simulink model "parallel_8_prediction_and_cost_function"  (R2022a)
settings: Solver=FixedStepDiscrete  StartTime=0.0  StopTime=10.0  RelTol=1e-3
undefined symbols (not defined in the file or in its folder): f_c, L_d, L_q, L_x, L_y, p, psi_pm, R_ph
libraries: hdlsllib x10
(part 2 of 2)

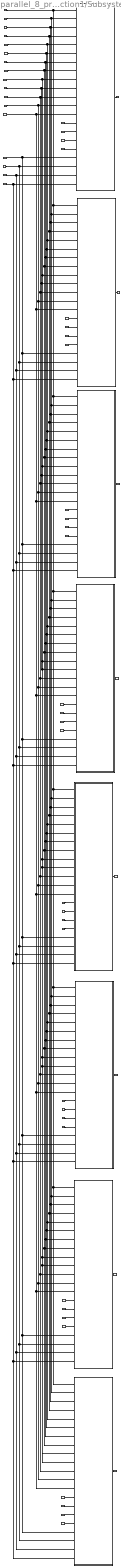
== system parallel_8_prediction_and_cost_function/Prediction_and_cost_function1/Subsystem ==
  d_phase_voltage_per_switching_state : Inport
  q_phase_voltage_per_switching_state : Inport  Port=2
  x_phase_voltage_per_switching_state : Inport  Port=3
  y_phase_voltage_per_switching_state : Inport  Port=4
  d_phase_voltage_per_switching_state1 : Inport  Port=5
  q_phase_voltage_per_switching_state1 : Inport  Port=6
  x_phase_voltage_per_switching_state1 : Inport  Port=7
  y_phase_voltage_per_switching_state1 : Inport  Port=8
  d_phase_voltage_per_switching_state2 : Inport  Port=9
  q_phase_voltage_per_switching_state2 : Inport  Port=10
  x_phase_voltage_per_switching_state2 : Inport  Port=11
  y_phase_voltage_per_switching_state2 : Inport  Port=12
  d_phase_voltage_per_switching_state3 : Inport  Port=13
  q_phase_voltage_per_switching_state3 : Inport  Port=14
  x_phase_voltage_per_switching_state3 : Inport  Port=15
  y_phase_voltage_per_switching_state3 : Inport  Port=16
  d_phase_voltage_per_switching_state4 : Inport  Port=17
  q_phase_voltage_per_switching_state4 : Inport  Port=18
  x_phase_voltage_per_switching_state4 : Inport  Port=19
  y_phase_voltage_per_switching_state4 : Inport  Port=20
  d_phase_voltage_per_switching_state5 : Inport  Port=21
  q_phase_voltage_per_switching_state5 : Inport  Port=22
  x_phase_voltage_per_switching_state5 : Inport  Port=23
  y_phase_voltage_per_switching_state5 : Inport  Port=24
  d_phase_voltage_per_switching_state6 : Inport  Port=25
  q_phase_voltage_per_switching_state6 : Inport  Port=26
  x_phase_voltage_per_switching_state6 : Inport  Port=27
  y_phase_voltage_per_switching_state6 : Inport  Port=28
  d_phase_voltage_per_switching_state7 : Inport  Port=29
  q_phase_voltage_per_switching_state7 : Inport  Port=30
  x_phase_voltage_per_switching_state7 : Inport  Port=31
  y_phase_voltage_per_switching_state7 : Inport  Port=32
  SampleTime_div_Ld15 : Inport  Port=33
  SampleTime_div_Lq15 : Inport  Port=34
  SampleTime_div_Lx15 : Inport  Port=35
  SampleTime_div_Ly15 : Inport  Port=36
  id_k_16 : Inport  Port=37
  iq_k_16 : Inport  Port=38
  ix_k_16 : Inport  Port=39
  iy_k_16 : Inport  Port=40
  Rs15 : Inport  Port=41
  omega_el15 : Inport  Port=42
  Lq15 : Inport  Port=43
  Ld15 : Inport  Port=44
  psiPM15 : Inport  Port=45
  id_ref15 : Inport  Port=46
  iq_ref15 : Inport  Port=47
  ix_ref15 : Inport  Port=48
  iy_ref15 : Inport  Port=49
  MATLAB Function10 : MATLAB Function  TreatAsAtomicUnit=on  SystemSampleTime=1/100000000
  MATLAB Function11 : MATLAB Function  TreatAsAtomicUnit=on  SystemSampleTime=1/100000000
  MATLAB Function12 : MATLAB Function  TreatAsAtomicUnit=on  SystemSampleTime=1/100000000
  MATLAB Function13 : MATLAB Function  TreatAsAtomicUnit=on  SystemSampleTime=1/100000000
  MATLAB Function14 : MATLAB Function  TreatAsAtomicUnit=on  SystemSampleTime=1/100000000
  MATLAB Function15 : MATLAB Function  TreatAsAtomicUnit=on  SystemSampleTime=1/100000000
  MATLAB Function8 : MATLAB Function  TreatAsAtomicUnit=on  SystemSampleTime=1/100000000
  MATLAB Function9 : MATLAB Function  TreatAsAtomicUnit=on  SystemSampleTime=1/100000000
  J : Outport
  J1 : Outport  Port=2
  J2 : Outport  Port=3
  J3 : Outport  Port=4
  J4 : Outport  Port=5
  J5 : Outport  Port=6
  J6 : Outport  Port=7
  J7 : Outport  Port=8
  wires:
  q_phase_voltage_per_switching_state1/1 -> MATLAB Function14/15(q_phase_voltage_per_switching_state)
  SampleTime_div_Ld15/1 -> MATLAB Function8/1(SampleTime_div_Ld), MATLAB Function9/1(SampleTime_div_Ld), MATLAB Function10/1(SampleTime_div_Ld), MATLAB Function11/1(SampleTime_div_Ld), MATLAB Function12/1(SampleTime_div_Ld), MATLAB Function13/1(SampleTime_div_Ld), MATLAB Function14/1(SampleTime_div_Ld), MATLAB Function15/1(SampleTime_div_Ld)
  Rs15/1 -> MATLAB Function8/9(Rs), MATLAB Function9/9(Rs), MATLAB Function10/9(Rs), MATLAB Function11/9(Rs), MATLAB Function12/9(Rs), MATLAB Function13/9(Rs), MATLAB Function14/9(Rs), MATLAB Function15/9(Rs)
  y_phase_voltage_per_switching_state/1 -> MATLAB Function15/17(y_phase_voltage_per_switching_state)
  Lq15/1 -> MATLAB Function8/11(Lq), MATLAB Function9/11(Lq), MATLAB Function10/11(Lq), MATLAB Function11/11(Lq), MATLAB Function12/11(Lq), MATLAB Function13/11(Lq), MATLAB Function14/11(Lq), MATLAB Function15/11(Lq)
  MATLAB Function11/1(J) -> J4/1
  y_phase_voltage_per_switching_state2/1 -> MATLAB Function13/17(y_phase_voltage_per_switching_state)
  d_phase_voltage_per_switching_state1/1 -> MATLAB Function14/14(d_phase_voltage_per_switching_state)
  x_phase_voltage_per_switching_state1/1 -> MATLAB Function14/16(x_phase_voltage_per_switching_state)
  y_phase_voltage_per_switching_state7/1 -> MATLAB Function8/17(y_phase_voltage_per_switching_state)
  iy_ref15/1 -> MATLAB Function8/21(iy_ref), MATLAB Function9/21(iy_ref), MATLAB Function10/21(iy_ref), MATLAB Function11/21(iy_ref), MATLAB Function12/21(iy_ref), MATLAB Function13/21(iy_ref), MATLAB Function14/21(iy_ref), MATLAB Function15/21(iy_ref)
  omega_el15/1 -> MATLAB Function8/10(omega_el), MATLAB Function9/10(omega_el), MATLAB Function10/10(omega_el), MATLAB Function11/10(omega_el), MATLAB Function12/10(omega_el), MATLAB Function13/10(omega_el), MATLAB Function14/10(omega_el), MATLAB Function15/10(omega_el)
  psiPM15/1 -> MATLAB Function8/13(psiPM), MATLAB Function9/13(psiPM), MATLAB Function10/13(psiPM), MATLAB Function11/13(psiPM), MATLAB Function12/13(psiPM), MATLAB Function13/13(psiPM), MATLAB Function14/13(psiPM), MATLAB Function15/13(psiPM)
  d_phase_voltage_per_switching_state3/1 -> MATLAB Function12/14(d_phase_voltage_per_switching_state)
  d_phase_voltage_per_switching_state6/1 -> MATLAB Function9/14(d_phase_voltage_per_switching_state)
  d_phase_voltage_per_switching_state/1 -> MATLAB Function15/14(d_phase_voltage_per_switching_state)
  x_phase_voltage_per_switching_state3/1 -> MATLAB Function12/16(x_phase_voltage_per_switching_state)
  d_phase_voltage_per_switching_state2/1 -> MATLAB Function13/14(d_phase_voltage_per_switching_state)
  x_phase_voltage_per_switching_state4/1 -> MATLAB Function11/16(x_phase_voltage_per_switching_state)
  y_phase_voltage_per_switching_state1/1 -> MATLAB Function14/17(y_phase_voltage_per_switching_state)
  MATLAB Function14/1(J) -> J1/1
  MATLAB Function8/1(J) -> J7/1
  q_phase_voltage_per_switching_state2/1 -> MATLAB Function13/15(q_phase_voltage_per_switching_state)
  x_phase_voltage_per_switching_state2/1 -> MATLAB Function13/16(x_phase_voltage_per_switching_state)
  MATLAB Function13/1(J) -> J2/1
  y_phase_voltage_per_switching_state4/1 -> MATLAB Function11/17(y_phase_voltage_per_switching_state)
  x_phase_voltage_per_switching_state/1 -> MATLAB Function15/16(x_phase_voltage_per_switching_state)
  q_phase_voltage_per_switching_state5/1 -> MATLAB Function10/15(q_phase_voltage_per_switching_state)
  d_phase_voltage_per_switching_state7/1 -> MATLAB Function8/14(d_phase_voltage_per_switching_state)
  d_phase_voltage_per_switching_state4/1 -> MATLAB Function11/14(d_phase_voltage_per_switching_state)
  q_phase_voltage_per_switching_state4/1 -> MATLAB Function11/15(q_phase_voltage_per_switching_state)
  x_phase_voltage_per_switching_state5/1 -> MATLAB Function10/16(x_phase_voltage_per_switching_state)
  SampleTime_div_Lx15/1 -> MATLAB Function8/3(SampleTime_div_Lx), MATLAB Function9/3(SampleTime_div_Lx), MATLAB Function10/3(SampleTime_div_Lx), MATLAB Function11/3(SampleTime_div_Lx), MATLAB Function12/3(SampleTime_div_Lx), MATLAB Function13/3(SampleTime_div_Lx), MATLAB Function14/3(SampleTime_div_Lx), MATLAB Function15/3(SampleTime_div_Lx)
  SampleTime_div_Ly15/1 -> MATLAB Function8/4(SampleTime_div_Ly), MATLAB Function9/4(SampleTime_div_Ly), MATLAB Function10/4(SampleTime_div_Ly), MATLAB Function11/4(SampleTime_div_Ly), MATLAB Function12/4(SampleTime_div_Ly), MATLAB Function13/4(SampleTime_div_Ly), MATLAB Function14/4(SampleTime_div_Ly), MATLAB Function15/4(SampleTime_div_Ly)
  SampleTime_div_Lq15/1 -> MATLAB Function8/2(SampleTime_div_Lq), MATLAB Function9/2(SampleTime_div_Lq), MATLAB Function10/2(SampleTime_div_Lq), MATLAB Function11/2(SampleTime_div_Lq), MATLAB Function12/2(SampleTime_div_Lq), MATLAB Function13/2(SampleTime_div_Lq), MATLAB Function14/2(SampleTime_div_Lq), MATLAB Function15/2(SampleTime_div_Lq)
  x_phase_voltage_per_switching_state7/1 -> MATLAB Function8/16(x_phase_voltage_per_switching_state)
  q_phase_voltage_per_switching_state/1 -> MATLAB Function15/15(q_phase_voltage_per_switching_state)
  MATLAB Function15/1(J) -> J/1
  d_phase_voltage_per_switching_state5/1 -> MATLAB Function10/14(d_phase_voltage_per_switching_state)
  MATLAB Function10/1(J) -> J5/1
  y_phase_voltage_per_switching_state5/1 -> MATLAB Function10/17(y_phase_voltage_per_switching_state)
  q_phase_voltage_per_switching_state6/1 -> MATLAB Function9/15(q_phase_voltage_per_switching_state)
  y_phase_voltage_per_switching_state6/1 -> MATLAB Function9/17(y_phase_voltage_per_switching_state)
  x_phase_voltage_per_switching_state6/1 -> MATLAB Function9/16(x_phase_voltage_per_switching_state)
  MATLAB Function9/1(J) -> J6/1
  MATLAB Function12/1(J) -> J3/1
  q_phase_voltage_per_switching_state7/1 -> MATLAB Function8/15(q_phase_voltage_per_switching_state)
  y_phase_voltage_per_switching_state3/1 -> MATLAB Function12/17(y_phase_voltage_per_switching_state)
  q_phase_voltage_per_switching_state3/1 -> MATLAB Function12/15(q_phase_voltage_per_switching_state)
  ix_ref15/1 -> MATLAB Function8/20(ix_ref), MATLAB Function9/20(ix_ref), MATLAB Function10/20(ix_ref), MATLAB Function11/20(ix_ref), MATLAB Function12/20(ix_ref), MATLAB Function13/20(ix_ref), MATLAB Function14/20(ix_ref), MATLAB Function15/20(ix_ref)
  iq_ref15/1 -> MATLAB Function8/19(iq_ref), MATLAB Function9/19(iq_ref), MATLAB Function10/19(iq_ref), MATLAB Function11/19(iq_ref), MATLAB Function12/19(iq_ref), MATLAB Function13/19(iq_ref), MATLAB Function14/19(iq_ref), MATLAB Function15/19(iq_ref)
  id_ref15/1 -> MATLAB Function8/18(id_ref), MATLAB Function9/18(id_ref), MATLAB Function10/18(id_ref), MATLAB Function11/18(id_ref), MATLAB Function12/18(id_ref), MATLAB Function13/18(id_ref), MATLAB Function14/18(id_ref), MATLAB Function15/18(id_ref)
  Ld15/1 -> MATLAB Function8/12(Ld), MATLAB Function9/12(Ld), MATLAB Function10/12(Ld), MATLAB Function11/12(Ld), MATLAB Function12/12(Ld), MATLAB Function13/12(Ld), MATLAB Function14/12(Ld), MATLAB Function15/12(Ld)
  iy_k_16/1 -> MATLAB Function8/8(iy_k_1), MATLAB Function9/8(iy_k_1), MATLAB Function10/8(iy_k_1), MATLAB Function11/8(iy_k_1), MATLAB Function12/8(iy_k_1), MATLAB Function13/8(iy_k_1), MATLAB Function14/8(iy_k_1), MATLAB Function15/8(iy_k_1)
  ix_k_16/1 -> MATLAB Function8/7(ix_k_1), MATLAB Function9/7(ix_k_1), MATLAB Function10/7(ix_k_1), MATLAB Function11/7(ix_k_1), MATLAB Function12/7(ix_k_1), MATLAB Function13/7(ix_k_1), MATLAB Function14/7(ix_k_1), MATLAB Function15/7(ix_k_1)
  iq_k_16/1 -> MATLAB Function8/6(iq_k_1), MATLAB Function9/6(iq_k_1), MATLAB Function10/6(iq_k_1), MATLAB Function11/6(iq_k_1), MATLAB Function12/6(iq_k_1), MATLAB Function13/6(iq_k_1), MATLAB Function14/6(iq_k_1), MATLAB Function15/6(iq_k_1)
  id_k_16/1 -> MATLAB Function8/5(id_k_1), MATLAB Function9/5(id_k_1), MATLAB Function10/5(id_k_1), MATLAB Function11/5(id_k_1), MATLAB Function12/5(id_k_1), MATLAB Function13/5(id_k_1), MATLAB Function14/5(id_k_1), MATLAB Function15/5(id_k_1)

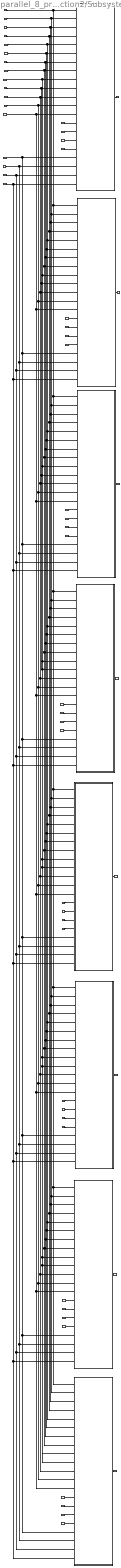
== system parallel_8_prediction_and_cost_function/Prediction_and_cost_function2/Subsystem ==
  d_phase_voltage_per_switching_state : Inport
  q_phase_voltage_per_switching_state : Inport  Port=2
  x_phase_voltage_per_switching_state : Inport  Port=3
  y_phase_voltage_per_switching_state : Inport  Port=4
  d_phase_voltage_per_switching_state1 : Inport  Port=5
  q_phase_voltage_per_switching_state1 : Inport  Port=6
  x_phase_voltage_per_switching_state1 : Inport  Port=7
  y_phase_voltage_per_switching_state1 : Inport  Port=8
  d_phase_voltage_per_switching_state2 : Inport  Port=9
  q_phase_voltage_per_switching_state2 : Inport  Port=10
  x_phase_voltage_per_switching_state2 : Inport  Port=11
  y_phase_voltage_per_switching_state2 : Inport  Port=12
  d_phase_voltage_per_switching_state3 : Inport  Port=13
  q_phase_voltage_per_switching_state3 : Inport  Port=14
  x_phase_voltage_per_switching_state3 : Inport  Port=15
  y_phase_voltage_per_switching_state3 : Inport  Port=16
  d_phase_voltage_per_switching_state4 : Inport  Port=17
  q_phase_voltage_per_switching_state4 : Inport  Port=18
  x_phase_voltage_per_switching_state4 : Inport  Port=19
  y_phase_voltage_per_switching_state4 : Inport  Port=20
  d_phase_voltage_per_switching_state5 : Inport  Port=21
  q_phase_voltage_per_switching_state5 : Inport  Port=22
  x_phase_voltage_per_switching_state5 : Inport  Port=23
  y_phase_voltage_per_switching_state5 : Inport  Port=24
  d_phase_voltage_per_switching_state6 : Inport  Port=25
  q_phase_voltage_per_switching_state6 : Inport  Port=26
  x_phase_voltage_per_switching_state6 : Inport  Port=27
  y_phase_voltage_per_switching_state6 : Inport  Port=28
  d_phase_voltage_per_switching_state7 : Inport  Port=29
  q_phase_voltage_per_switching_state7 : Inport  Port=30
  x_phase_voltage_per_switching_state7 : Inport  Port=31
  y_phase_voltage_per_switching_state7 : Inport  Port=32
  SampleTime_div_Ld15 : Inport  Port=33
  SampleTime_div_Lq15 : Inport  Port=34
  SampleTime_div_Lx15 : Inport  Port=35
  SampleTime_div_Ly15 : Inport  Port=36
  id_k_16 : Inport  Port=37
  iq_k_16 : Inport  Port=38
  ix_k_16 : Inport  Port=39
  iy_k_16 : Inport  Port=40
  Rs15 : Inport  Port=41
  omega_el15 : Inport  Port=42
  Lq15 : Inport  Port=43
  Ld15 : Inport  Port=44
  psiPM15 : Inport  Port=45
  id_ref15 : Inport  Port=46
  iq_ref15 : Inport  Port=47
  ix_ref15 : Inport  Port=48
  iy_ref15 : Inport  Port=49
  MATLAB Function10 : MATLAB Function  TreatAsAtomicUnit=on  SystemSampleTime=1/100000000
  MATLAB Function11 : MATLAB Function  TreatAsAtomicUnit=on  SystemSampleTime=1/100000000
  MATLAB Function12 : MATLAB Function  TreatAsAtomicUnit=on  SystemSampleTime=1/100000000
  MATLAB Function13 : MATLAB Function  TreatAsAtomicUnit=on  SystemSampleTime=1/100000000
  MATLAB Function14 : MATLAB Function  TreatAsAtomicUnit=on  SystemSampleTime=1/100000000
  MATLAB Function15 : MATLAB Function  TreatAsAtomicUnit=on  SystemSampleTime=1/100000000
  MATLAB Function8 : MATLAB Function  TreatAsAtomicUnit=on  SystemSampleTime=1/100000000
  MATLAB Function9 : MATLAB Function  TreatAsAtomicUnit=on  SystemSampleTime=1/100000000
  J : Outport
  J1 : Outport  Port=2
  J2 : Outport  Port=3
  J3 : Outport  Port=4
  J4 : Outport  Port=5
  J5 : Outport  Port=6
  J6 : Outport  Port=7
  J7 : Outport  Port=8
  wires:
  q_phase_voltage_per_switching_state1/1 -> MATLAB Function14/15(q_phase_voltage_per_switching_state)
  SampleTime_div_Ld15/1 -> MATLAB Function8/1(SampleTime_div_Ld), MATLAB Function9/1(SampleTime_div_Ld), MATLAB Function10/1(SampleTime_div_Ld), MATLAB Function11/1(SampleTime_div_Ld), MATLAB Function12/1(SampleTime_div_Ld), MATLAB Function13/1(SampleTime_div_Ld), MATLAB Function14/1(SampleTime_div_Ld), MATLAB Function15/1(SampleTime_div_Ld)
  Rs15/1 -> MATLAB Function8/9(Rs), MATLAB Function9/9(Rs), MATLAB Function10/9(Rs), MATLAB Function11/9(Rs), MATLAB Function12/9(Rs), MATLAB Function13/9(Rs), MATLAB Function14/9(Rs), MATLAB Function15/9(Rs)
  y_phase_voltage_per_switching_state/1 -> MATLAB Function15/17(y_phase_voltage_per_switching_state)
  Lq15/1 -> MATLAB Function8/11(Lq), MATLAB Function9/11(Lq), MATLAB Function10/11(Lq), MATLAB Function11/11(Lq), MATLAB Function12/11(Lq), MATLAB Function13/11(Lq), MATLAB Function14/11(Lq), MATLAB Function15/11(Lq)
  MATLAB Function11/1(J) -> J4/1
  y_phase_voltage_per_switching_state2/1 -> MATLAB Function13/17(y_phase_voltage_per_switching_state)
  d_phase_voltage_per_switching_state1/1 -> MATLAB Function14/14(d_phase_voltage_per_switching_state)
  x_phase_voltage_per_switching_state1/1 -> MATLAB Function14/16(x_phase_voltage_per_switching_state)
  y_phase_voltage_per_switching_state7/1 -> MATLAB Function8/17(y_phase_voltage_per_switching_state)
  iy_ref15/1 -> MATLAB Function8/21(iy_ref), MATLAB Function9/21(iy_ref), MATLAB Function10/21(iy_ref), MATLAB Function11/21(iy_ref), MATLAB Function12/21(iy_ref), MATLAB Function13/21(iy_ref), MATLAB Function14/21(iy_ref), MATLAB Function15/21(iy_ref)
  omega_el15/1 -> MATLAB Function8/10(omega_el), MATLAB Function9/10(omega_el), MATLAB Function10/10(omega_el), MATLAB Function11/10(omega_el), MATLAB Function12/10(omega_el), MATLAB Function13/10(omega_el), MATLAB Function14/10(omega_el), MATLAB Function15/10(omega_el)
  psiPM15/1 -> MATLAB Function8/13(psiPM), MATLAB Function9/13(psiPM), MATLAB Function10/13(psiPM), MATLAB Function11/13(psiPM), MATLAB Function12/13(psiPM), MATLAB Function13/13(psiPM), MATLAB Function14/13(psiPM), MATLAB Function15/13(psiPM)
  d_phase_voltage_per_switching_state3/1 -> MATLAB Function12/14(d_phase_voltage_per_switching_state)
  d_phase_voltage_per_switching_state6/1 -> MATLAB Function9/14(d_phase_voltage_per_switching_state)
  d_phase_voltage_per_switching_state/1 -> MATLAB Function15/14(d_phase_voltage_per_switching_state)
  x_phase_voltage_per_switching_state3/1 -> MATLAB Function12/16(x_phase_voltage_per_switching_state)
  d_phase_voltage_per_switching_state2/1 -> MATLAB Function13/14(d_phase_voltage_per_switching_state)
  x_phase_voltage_per_switching_state4/1 -> MATLAB Function11/16(x_phase_voltage_per_switching_state)
  y_phase_voltage_per_switching_state1/1 -> MATLAB Function14/17(y_phase_voltage_per_switching_state)
  MATLAB Function14/1(J) -> J1/1
  MATLAB Function8/1(J) -> J7/1
  q_phase_voltage_per_switching_state2/1 -> MATLAB Function13/15(q_phase_voltage_per_switching_state)
  x_phase_voltage_per_switching_state2/1 -> MATLAB Function13/16(x_phase_voltage_per_switching_state)
  MATLAB Function13/1(J) -> J2/1
  y_phase_voltage_per_switching_state4/1 -> MATLAB Function11/17(y_phase_voltage_per_switching_state)
  x_phase_voltage_per_switching_state/1 -> MATLAB Function15/16(x_phase_voltage_per_switching_state)
  q_phase_voltage_per_switching_state5/1 -> MATLAB Function10/15(q_phase_voltage_per_switching_state)
  d_phase_voltage_per_switching_state7/1 -> MATLAB Function8/14(d_phase_voltage_per_switching_state)
  d_phase_voltage_per_switching_state4/1 -> MATLAB Function11/14(d_phase_voltage_per_switching_state)
  q_phase_voltage_per_switching_state4/1 -> MATLAB Function11/15(q_phase_voltage_per_switching_state)
  x_phase_voltage_per_switching_state5/1 -> MATLAB Function10/16(x_phase_voltage_per_switching_state)
  SampleTime_div_Lx15/1 -> MATLAB Function8/3(SampleTime_div_Lx), MATLAB Function9/3(SampleTime_div_Lx), MATLAB Function10/3(SampleTime_div_Lx), MATLAB Function11/3(SampleTime_div_Lx), MATLAB Function12/3(SampleTime_div_Lx), MATLAB Function13/3(SampleTime_div_Lx), MATLAB Function14/3(SampleTime_div_Lx), MATLAB Function15/3(SampleTime_div_Lx)
  SampleTime_div_Ly15/1 -> MATLAB Function8/4(SampleTime_div_Ly), MATLAB Function9/4(SampleTime_div_Ly), MATLAB Function10/4(SampleTime_div_Ly), MATLAB Function11/4(SampleTime_div_Ly), MATLAB Function12/4(SampleTime_div_Ly), MATLAB Function13/4(SampleTime_div_Ly), MATLAB Function14/4(SampleTime_div_Ly), MATLAB Function15/4(SampleTime_div_Ly)
  SampleTime_div_Lq15/1 -> MATLAB Function8/2(SampleTime_div_Lq), MATLAB Function9/2(SampleTime_div_Lq), MATLAB Function10/2(SampleTime_div_Lq), MATLAB Function11/2(SampleTime_div_Lq), MATLAB Function12/2(SampleTime_div_Lq), MATLAB Function13/2(SampleTime_div_Lq), MATLAB Function14/2(SampleTime_div_Lq), MATLAB Function15/2(SampleTime_div_Lq)
  x_phase_voltage_per_switching_state7/1 -> MATLAB Function8/16(x_phase_voltage_per_switching_state)
  q_phase_voltage_per_switching_state/1 -> MATLAB Function15/15(q_phase_voltage_per_switching_state)
  MATLAB Function15/1(J) -> J/1
  d_phase_voltage_per_switching_state5/1 -> MATLAB Function10/14(d_phase_voltage_per_switching_state)
  MATLAB Function10/1(J) -> J5/1
  y_phase_voltage_per_switching_state5/1 -> MATLAB Function10/17(y_phase_voltage_per_switching_state)
  q_phase_voltage_per_switching_state6/1 -> MATLAB Function9/15(q_phase_voltage_per_switching_state)
  y_phase_voltage_per_switching_state6/1 -> MATLAB Function9/17(y_phase_voltage_per_switching_state)
  x_phase_voltage_per_switching_state6/1 -> MATLAB Function9/16(x_phase_voltage_per_switching_state)
  MATLAB Function9/1(J) -> J6/1
  MATLAB Function12/1(J) -> J3/1
  q_phase_voltage_per_switching_state7/1 -> MATLAB Function8/15(q_phase_voltage_per_switching_state)
  y_phase_voltage_per_switching_state3/1 -> MATLAB Function12/17(y_phase_voltage_per_switching_state)
  q_phase_voltage_per_switching_state3/1 -> MATLAB Function12/15(q_phase_voltage_per_switching_state)
  ix_ref15/1 -> MATLAB Function8/20(ix_ref), MATLAB Function9/20(ix_ref), MATLAB Function10/20(ix_ref), MATLAB Function11/20(ix_ref), MATLAB Function12/20(ix_ref), MATLAB Function13/20(ix_ref), MATLAB Function14/20(ix_ref), MATLAB Function15/20(ix_ref)
  iq_ref15/1 -> MATLAB Function8/19(iq_ref), MATLAB Function9/19(iq_ref), MATLAB Function10/19(iq_ref), MATLAB Function11/19(iq_ref), MATLAB Function12/19(iq_ref), MATLAB Function13/19(iq_ref), MATLAB Function14/19(iq_ref), MATLAB Function15/19(iq_ref)
  id_ref15/1 -> MATLAB Function8/18(id_ref), MATLAB Function9/18(id_ref), MATLAB Function10/18(id_ref), MATLAB Function11/18(id_ref), MATLAB Function12/18(id_ref), MATLAB Function13/18(id_ref), MATLAB Function14/18(id_ref), MATLAB Function15/18(id_ref)
  Ld15/1 -> MATLAB Function8/12(Ld), MATLAB Function9/12(Ld), MATLAB Function10/12(Ld), MATLAB Function11/12(Ld), MATLAB Function12/12(Ld), MATLAB Function13/12(Ld), MATLAB Function14/12(Ld), MATLAB Function15/12(Ld)
  iy_k_16/1 -> MATLAB Function8/8(iy_k_1), MATLAB Function9/8(iy_k_1), MATLAB Function10/8(iy_k_1), MATLAB Function11/8(iy_k_1), MATLAB Function12/8(iy_k_1), MATLAB Function13/8(iy_k_1), MATLAB Function14/8(iy_k_1), MATLAB Function15/8(iy_k_1)
  ix_k_16/1 -> MATLAB Function8/7(ix_k_1), MATLAB Function9/7(ix_k_1), MATLAB Function10/7(ix_k_1), MATLAB Function11/7(ix_k_1), MATLAB Function12/7(ix_k_1), MATLAB Function13/7(ix_k_1), MATLAB Function14/7(ix_k_1), MATLAB Function15/7(ix_k_1)
  iq_k_16/1 -> MATLAB Function8/6(iq_k_1), MATLAB Function9/6(iq_k_1), MATLAB Function10/6(iq_k_1), MATLAB Function11/6(iq_k_1), MATLAB Function12/6(iq_k_1), MATLAB Function13/6(iq_k_1), MATLAB Function14/6(iq_k_1), MATLAB Function15/6(iq_k_1)
  id_k_16/1 -> MATLAB Function8/5(id_k_1), MATLAB Function9/5(id_k_1), MATLAB Function10/5(id_k_1), MATLAB Function11/5(id_k_1), MATLAB Function12/5(id_k_1), MATLAB Function13/5(id_k_1), MATLAB Function14/5(id_k_1), MATLAB Function15/5(id_k_1)

== matlab function parallel_8_prediction_and_cost_function/Prediction_and_cost_function1/Subsystem/MATLAB Function13 ==
  data: SampleTime_div_Ld input; J output; SampleTime_div_Lq input; SampleTime_div_Lx input; SampleTime_div_Ly input; id_k_1 input; iq_k_1 input; ix_k_1 input; iy_k_1 input; Rs input; omega_el input; Lq input; Ld input; psiPM input; d_phase_voltage_per_switching_state input; q_phase_voltage_per_switching_state input; x_phase_voltage_per_switching_state input; y_phase_voltage_per_switching_state input; id_ref input; iq_ref input; ix_ref input; iy_ref input
function J = fcn(SampleTime_div_Ld, SampleTime_div_Lq, SampleTime_div_Lx, SampleTime_div_Ly, id_k_1, iq_k_1, ix_k_1, iy_k_1, Rs, omega_el, Lq, Ld, psiPM, d_phase_voltage_per_switching_state, q_phase_voltage_per_switching_state, x_phase_voltage_per_switching_state, y_phase_voltage_per_switching_state, id_ref, iq_ref, ix_ref, iy_ref)
     
        % Prediction of the d-, q-, x-, y-currents of the 6-Phase-PMSM with the finite control set 
        id_k_2 = single(SampleTime_div_Ld*(d_phase_voltage_per_switching_state-id_k_1*Rs+omega_el*Lq*iq_k_1)+id_k_1);
        iq_k_2 = single(SampleTime_div_Lq*(q_phase_voltage_per_switching_state-iq_k_1*Rs-omega_el*(psiPM+id_k_1*Ld))+iq_k_1);
        ix_k_2 = single(SampleTime_div_Lx*(x_phase_voltage_per_switching_state-ix_k_1*Rs)+ix_k_1);
        iy_k_2 = single(SampleTime_div_Ly*(y_phase_voltage_per_switching_state-iy_k_1*Rs)+iy_k_1);
        
        % Calculation of the cost function
        J = single((id_ref-id_k_2)^2+(iq_ref-iq_k_2)^2+(ix_ref-ix_k_2)^2+(iy_ref-iy_k_2)^2);

end

== matlab function parallel_8_prediction_and_cost_function/Prediction_and_cost_function1/Subsystem/MATLAB Function14 ==
  data: SampleTime_div_Ld input; J output; SampleTime_div_Lq input; SampleTime_div_Lx input; SampleTime_div_Ly input; id_k_1 input; iq_k_1 input; ix_k_1 input; iy_k_1 input; Rs input; omega_el input; Lq input; Ld input; psiPM input; d_phase_voltage_per_switching_state input; q_phase_voltage_per_switching_state input; x_phase_voltage_per_switching_state input; y_phase_voltage_per_switching_state input; id_ref input; iq_ref input; ix_ref input; iy_ref input
function J = fcn(SampleTime_div_Ld, SampleTime_div_Lq, SampleTime_div_Lx, SampleTime_div_Ly, id_k_1, iq_k_1, ix_k_1, iy_k_1, Rs, omega_el, Lq, Ld, psiPM, d_phase_voltage_per_switching_state, q_phase_voltage_per_switching_state, x_phase_voltage_per_switching_state, y_phase_voltage_per_switching_state, id_ref, iq_ref, ix_ref, iy_ref)
     
        % Prediction of the d-, q-, x-, y-currents of the 6-Phase-PMSM with the finite control set 
        id_k_2 = single(SampleTime_div_Ld*(d_phase_voltage_per_switching_state-id_k_1*Rs+omega_el*Lq*iq_k_1)+id_k_1);
        iq_k_2 = single(SampleTime_div_Lq*(q_phase_voltage_per_switching_state-iq_k_1*Rs-omega_el*(psiPM+id_k_1*Ld))+iq_k_1);
        ix_k_2 = single(SampleTime_div_Lx*(x_phase_voltage_per_switching_state-ix_k_1*Rs)+ix_k_1);
        iy_k_2 = single(SampleTime_div_Ly*(y_phase_voltage_per_switching_state-iy_k_1*Rs)+iy_k_1);
        
        % Calculation of the cost function
        J = single((id_ref-id_k_2)^2+(iq_ref-iq_k_2)^2+(ix_ref-ix_k_2)^2+(iy_ref-iy_k_2)^2);
      

end

== matlab function parallel_8_prediction_and_cost_function/Prediction_and_cost_function1/Subsystem/MATLAB Function15 ==
  data: SampleTime_div_Ld input; J output; SampleTime_div_Lq input; SampleTime_div_Lx input; SampleTime_div_Ly input; id_k_1 input; iq_k_1 input; ix_k_1 input; iy_k_1 input; Rs input; omega_el input; Lq input; Ld input; psiPM input; d_phase_voltage_per_switching_state input; q_phase_voltage_per_switching_state input; x_phase_voltage_per_switching_state input; y_phase_voltage_per_switching_state input; id_ref input; iq_ref input; ix_ref input; iy_ref input
function J = fcn(SampleTime_div_Ld, SampleTime_div_Lq, SampleTime_div_Lx, SampleTime_div_Ly, id_k_1, iq_k_1, ix_k_1, iy_k_1, Rs, omega_el, Lq, Ld, psiPM, d_phase_voltage_per_switching_state, q_phase_voltage_per_switching_state, x_phase_voltage_per_switching_state, y_phase_voltage_per_switching_state, id_ref, iq_ref, ix_ref, iy_ref)
     
        % Prediction of the d-, q-, x-, y-currents of the 6-Phase-PMSM with the finite control set 
        id_k_2 = single(SampleTime_div_Ld*(d_phase_voltage_per_switching_state-id_k_1*Rs+omega_el*Lq*iq_k_1)+id_k_1);
        iq_k_2 = single(SampleTime_div_Lq*(q_phase_voltage_per_switching_state-iq_k_1*Rs-omega_el*(psiPM+id_k_1*Ld))+iq_k_1);
        ix_k_2 = single(SampleTime_div_Lx*(x_phase_voltage_per_switching_state-ix_k_1*Rs)+ix_k_1);
        iy_k_2 = single(SampleTime_div_Ly*(y_phase_voltage_per_switching_state-iy_k_1*Rs)+iy_k_1);
        
        % Calculation of the cost function
        J = single((id_ref-id_k_2)^2+(iq_ref-iq_k_2)^2+(ix_ref-ix_k_2)^2+(iy_ref-iy_k_2)^2);

end

== matlab function parallel_8_prediction_and_cost_function/Prediction_and_cost_function1/Subsystem/MATLAB Function8 ==
  data: SampleTime_div_Ld input; J output; SampleTime_div_Lq input; SampleTime_div_Lx input; SampleTime_div_Ly input; id_k_1 input; iq_k_1 input; ix_k_1 input; iy_k_1 input; Rs input; omega_el input; Lq input; Ld input; psiPM input; d_phase_voltage_per_switching_state input; q_phase_voltage_per_switching_state input; x_phase_voltage_per_switching_state input; y_phase_voltage_per_switching_state input; id_ref input; iq_ref input; ix_ref input; iy_ref input
function J = fcn(SampleTime_div_Ld, SampleTime_div_Lq, SampleTime_div_Lx, SampleTime_div_Ly, id_k_1, iq_k_1, ix_k_1, iy_k_1, Rs, omega_el, Lq, Ld, psiPM, d_phase_voltage_per_switching_state, q_phase_voltage_per_switching_state, x_phase_voltage_per_switching_state, y_phase_voltage_per_switching_state, id_ref, iq_ref, ix_ref, iy_ref)
     
        % Prediction of the d-, q-, x-, y-currents of the 6-Phase-PMSM with the finite control set 
        id_k_2 = single(SampleTime_div_Ld*(d_phase_voltage_per_switching_state-id_k_1*Rs+omega_el*Lq*iq_k_1)+id_k_1);
        iq_k_2 = single(SampleTime_div_Lq*(q_phase_voltage_per_switching_state-iq_k_1*Rs-omega_el*(psiPM+id_k_1*Ld))+iq_k_1);
        ix_k_2 = single(SampleTime_div_Lx*(x_phase_voltage_per_switching_state-ix_k_1*Rs)+ix_k_1);
        iy_k_2 = single(SampleTime_div_Ly*(y_phase_voltage_per_switching_state-iy_k_1*Rs)+iy_k_1);
        
        % Calculation of the cost function
        J = single((id_ref-id_k_2)^2+(iq_ref-iq_k_2)^2+(ix_ref-ix_k_2)^2+(iy_ref-iy_k_2)^2);

end

== matlab function parallel_8_prediction_and_cost_function/Prediction_and_cost_function1/Subsystem/MATLAB Function9 ==
  data: SampleTime_div_Ld input; J output; SampleTime_div_Lq input; SampleTime_div_Lx input; SampleTime_div_Ly input; id_k_1 input; iq_k_1 input; ix_k_1 input; iy_k_1 input; Rs input; omega_el input; Lq input; Ld input; psiPM input; d_phase_voltage_per_switching_state input; q_phase_voltage_per_switching_state input; x_phase_voltage_per_switching_state input; y_phase_voltage_per_switching_state input; id_ref input; iq_ref input; ix_ref input; iy_ref input
function J = fcn(SampleTime_div_Ld, SampleTime_div_Lq, SampleTime_div_Lx, SampleTime_div_Ly, id_k_1, iq_k_1, ix_k_1, iy_k_1, Rs, omega_el, Lq, Ld, psiPM, d_phase_voltage_per_switching_state, q_phase_voltage_per_switching_state, x_phase_voltage_per_switching_state, y_phase_voltage_per_switching_state, id_ref, iq_ref, ix_ref, iy_ref)
     
        % Prediction of the d-, q-, x-, y-currents of the 6-Phase-PMSM with the finite control set 
        id_k_2 = single(SampleTime_div_Ld*(d_phase_voltage_per_switching_state-id_k_1*Rs+omega_el*Lq*iq_k_1)+id_k_1);
        iq_k_2 = single(SampleTime_div_Lq*(q_phase_voltage_per_switching_state-iq_k_1*Rs-omega_el*(psiPM+id_k_1*Ld))+iq_k_1);
        ix_k_2 = single(SampleTime_div_Lx*(x_phase_voltage_per_switching_state-ix_k_1*Rs)+ix_k_1);
        iy_k_2 = single(SampleTime_div_Ly*(y_phase_voltage_per_switching_state-iy_k_1*Rs)+iy_k_1);
        
        % Calculation of the cost function
        J = single((id_ref-id_k_2)^2+(iq_ref-iq_k_2)^2+(ix_ref-ix_k_2)^2+(iy_ref-iy_k_2)^2);

end

== matlab function parallel_8_prediction_and_cost_function/Prediction_and_cost_function2/Subsystem/MATLAB Function10 ==
  data: SampleTime_div_Ld input; J output; SampleTime_div_Lq input; SampleTime_div_Lx input; SampleTime_div_Ly input; id_k_1 input; iq_k_1 input; ix_k_1 input; iy_k_1 input; Rs input; omega_el input; Lq input; Ld input; psiPM input; d_phase_voltage_per_switching_state input; q_phase_voltage_per_switching_state input; x_phase_voltage_per_switching_state input; y_phase_voltage_per_switching_state input; id_ref input; iq_ref input; ix_ref input; iy_ref input
function J = fcn(SampleTime_div_Ld, SampleTime_div_Lq, SampleTime_div_Lx, SampleTime_div_Ly, id_k_1, iq_k_1, ix_k_1, iy_k_1, Rs, omega_el, Lq, Ld, psiPM, d_phase_voltage_per_switching_state, q_phase_voltage_per_switching_state, x_phase_voltage_per_switching_state, y_phase_voltage_per_switching_state, id_ref, iq_ref, ix_ref, iy_ref)
     
        % Prediction of the d-, q-, x-, y-currents of the 6-Phase-PMSM with the finite control set 
        id_k_2 = single(SampleTime_div_Ld*(d_phase_voltage_per_switching_state-id_k_1*Rs+omega_el*Lq*iq_k_1)+id_k_1);
        iq_k_2 = single(SampleTime_div_Lq*(q_phase_voltage_per_switching_state-iq_k_1*Rs-omega_el*(psiPM+id_k_1*Ld))+iq_k_1);
        ix_k_2 = single(SampleTime_div_Lx*(x_phase_voltage_per_switching_state-ix_k_1*Rs)+ix_k_1);
        iy_k_2 = single(SampleTime_div_Ly*(y_phase_voltage_per_switching_state-iy_k_1*Rs)+iy_k_1);
        
        % Calculation of the cost function
        J = single((id_ref-id_k_2)^2+(iq_ref-iq_k_2)^2+(ix_ref-ix_k_2)^2+(iy_ref-iy_k_2)^2);

end

== matlab function parallel_8_prediction_and_cost_function/Prediction_and_cost_function1/Subsystem/MATLAB Function10 ==
  data: SampleTime_div_Ld input; J output; SampleTime_div_Lq input; SampleTime_div_Lx input; SampleTime_div_Ly input; id_k_1 input; iq_k_1 input; ix_k_1 input; iy_k_1 input; Rs input; omega_el input; Lq input; Ld input; psiPM input; d_phase_voltage_per_switching_state input; q_phase_voltage_per_switching_state input; x_phase_voltage_per_switching_state input; y_phase_voltage_per_switching_state input; id_ref input; iq_ref input; ix_ref input; iy_ref input
function J = fcn(SampleTime_div_Ld, SampleTime_div_Lq, SampleTime_div_Lx, SampleTime_div_Ly, id_k_1, iq_k_1, ix_k_1, iy_k_1, Rs, omega_el, Lq, Ld, psiPM, d_phase_voltage_per_switching_state, q_phase_voltage_per_switching_state, x_phase_voltage_per_switching_state, y_phase_voltage_per_switching_state, id_ref, iq_ref, ix_ref, iy_ref)
     
        % Prediction of the d-, q-, x-, y-currents of the 6-Phase-PMSM with the finite control set 
        id_k_2 = single(SampleTime_div_Ld*(d_phase_voltage_per_switching_state-id_k_1*Rs+omega_el*Lq*iq_k_1)+id_k_1);
        iq_k_2 = single(SampleTime_div_Lq*(q_phase_voltage_per_switching_state-iq_k_1*Rs-omega_el*(psiPM+id_k_1*Ld))+iq_k_1);
        ix_k_2 = single(SampleTime_div_Lx*(x_phase_voltage_per_switching_state-ix_k_1*Rs)+ix_k_1);
        iy_k_2 = single(SampleTime_div_Ly*(y_phase_voltage_per_switching_state-iy_k_1*Rs)+iy_k_1);
        
        % Calculation of the cost function
        J = single((id_ref-id_k_2)^2+(iq_ref-iq_k_2)^2+(ix_ref-ix_k_2)^2+(iy_ref-iy_k_2)^2);

end

== matlab function parallel_8_prediction_and_cost_function/Prediction_and_cost_function2/Subsystem/MATLAB Function11 ==
  data: SampleTime_div_Ld input; J output; SampleTime_div_Lq input; SampleTime_div_Lx input; SampleTime_div_Ly input; id_k_1 input; iq_k_1 input; ix_k_1 input; iy_k_1 input; Rs input; omega_el input; Lq input; Ld input; psiPM input; d_phase_voltage_per_switching_state input; q_phase_voltage_per_switching_state input; x_phase_voltage_per_switching_state input; y_phase_voltage_per_switching_state input; id_ref input; iq_ref input; ix_ref input; iy_ref input
function J = fcn(SampleTime_div_Ld, SampleTime_div_Lq, SampleTime_div_Lx, SampleTime_div_Ly, id_k_1, iq_k_1, ix_k_1, iy_k_1, Rs, omega_el, Lq, Ld, psiPM, d_phase_voltage_per_switching_state, q_phase_voltage_per_switching_state, x_phase_voltage_per_switching_state, y_phase_voltage_per_switching_state, id_ref, iq_ref, ix_ref, iy_ref)
     
        % Prediction of the d-, q-, x-, y-currents of the 6-Phase-PMSM with the finite control set 
        id_k_2 = single(SampleTime_div_Ld*(d_phase_voltage_per_switching_state-id_k_1*Rs+omega_el*Lq*iq_k_1)+id_k_1);
        iq_k_2 = single(SampleTime_div_Lq*(q_phase_voltage_per_switching_state-iq_k_1*Rs-omega_el*(psiPM+id_k_1*Ld))+iq_k_1);
        ix_k_2 = single(SampleTime_div_Lx*(x_phase_voltage_per_switching_state-ix_k_1*Rs)+ix_k_1);
        iy_k_2 = single(SampleTime_div_Ly*(y_phase_voltage_per_switching_state-iy_k_1*Rs)+iy_k_1);
        
        % Calculation of the cost function
        J = single((id_ref-id_k_2)^2+(iq_ref-iq_k_2)^2+(ix_ref-ix_k_2)^2+(iy_ref-iy_k_2)^2);

end

== matlab function parallel_8_prediction_and_cost_function/Prediction_and_cost_function2/Subsystem/MATLAB Function12 ==
  data: SampleTime_div_Ld input; J output; SampleTime_div_Lq input; SampleTime_div_Lx input; SampleTime_div_Ly input; id_k_1 input; iq_k_1 input; ix_k_1 input; iy_k_1 input; Rs input; omega_el input; Lq input; Ld input; psiPM input; d_phase_voltage_per_switching_state input; q_phase_voltage_per_switching_state input; x_phase_voltage_per_switching_state input; y_phase_voltage_per_switching_state input; id_ref input; iq_ref input; ix_ref input; iy_ref input
function J = fcn(SampleTime_div_Ld, SampleTime_div_Lq, SampleTime_div_Lx, SampleTime_div_Ly, id_k_1, iq_k_1, ix_k_1, iy_k_1, Rs, omega_el, Lq, Ld, psiPM, d_phase_voltage_per_switching_state, q_phase_voltage_per_switching_state, x_phase_voltage_per_switching_state, y_phase_voltage_per_switching_state, id_ref, iq_ref, ix_ref, iy_ref)
     
        % Prediction of the d-, q-, x-, y-currents of the 6-Phase-PMSM with the finite control set 
        id_k_2 = single(SampleTime_div_Ld*(d_phase_voltage_per_switching_state-id_k_1*Rs+omega_el*Lq*iq_k_1)+id_k_1);
        iq_k_2 = single(SampleTime_div_Lq*(q_phase_voltage_per_switching_state-iq_k_1*Rs-omega_el*(psiPM+id_k_1*Ld))+iq_k_1);
        ix_k_2 = single(SampleTime_div_Lx*(x_phase_voltage_per_switching_state-ix_k_1*Rs)+ix_k_1);
        iy_k_2 = single(SampleTime_div_Ly*(y_phase_voltage_per_switching_state-iy_k_1*Rs)+iy_k_1);
        
        % Calculation of the cost function
        J = single((id_ref-id_k_2)^2+(iq_ref-iq_k_2)^2+(ix_ref-ix_k_2)^2+(iy_ref-iy_k_2)^2);

end

== matlab function parallel_8_prediction_and_cost_function/Prediction_and_cost_function2/Subsystem/MATLAB Function13 ==
  data: SampleTime_div_Ld input; J output; SampleTime_div_Lq input; SampleTime_div_Lx input; SampleTime_div_Ly input; id_k_1 input; iq_k_1 input; ix_k_1 input; iy_k_1 input; Rs input; omega_el input; Lq input; Ld input; psiPM input; d_phase_voltage_per_switching_state input; q_phase_voltage_per_switching_state input; x_phase_voltage_per_switching_state input; y_phase_voltage_per_switching_state input; id_ref input; iq_ref input; ix_ref input; iy_ref input
function J = fcn(SampleTime_div_Ld, SampleTime_div_Lq, SampleTime_div_Lx, SampleTime_div_Ly, id_k_1, iq_k_1, ix_k_1, iy_k_1, Rs, omega_el, Lq, Ld, psiPM, d_phase_voltage_per_switching_state, q_phase_voltage_per_switching_state, x_phase_voltage_per_switching_state, y_phase_voltage_per_switching_state, id_ref, iq_ref, ix_ref, iy_ref)
     
        % Prediction of the d-, q-, x-, y-currents of the 6-Phase-PMSM with the finite control set 
        id_k_2 = single(SampleTime_div_Ld*(d_phase_voltage_per_switching_state-id_k_1*Rs+omega_el*Lq*iq_k_1)+id_k_1);
        iq_k_2 = single(SampleTime_div_Lq*(q_phase_voltage_per_switching_state-iq_k_1*Rs-omega_el*(psiPM+id_k_1*Ld))+iq_k_1);
        ix_k_2 = single(SampleTime_div_Lx*(x_phase_voltage_per_switching_state-ix_k_1*Rs)+ix_k_1);
        iy_k_2 = single(SampleTime_div_Ly*(y_phase_voltage_per_switching_state-iy_k_1*Rs)+iy_k_1);
        
        % Calculation of the cost function
        J = single((id_ref-id_k_2)^2+(iq_ref-iq_k_2)^2+(ix_ref-ix_k_2)^2+(iy_ref-iy_k_2)^2);

end

== matlab function parallel_8_prediction_and_cost_function/Prediction_and_cost_function2/Subsystem/MATLAB Function14 ==
  data: SampleTime_div_Ld input; J output; SampleTime_div_Lq input; SampleTime_div_Lx input; SampleTime_div_Ly input; id_k_1 input; iq_k_1 input; ix_k_1 input; iy_k_1 input; Rs input; omega_el input; Lq input; Ld input; psiPM input; d_phase_voltage_per_switching_state input; q_phase_voltage_per_switching_state input; x_phase_voltage_per_switching_state input; y_phase_voltage_per_switching_state input; id_ref input; iq_ref input; ix_ref input; iy_ref input
function J = fcn(SampleTime_div_Ld, SampleTime_div_Lq, SampleTime_div_Lx, SampleTime_div_Ly, id_k_1, iq_k_1, ix_k_1, iy_k_1, Rs, omega_el, Lq, Ld, psiPM, d_phase_voltage_per_switching_state, q_phase_voltage_per_switching_state, x_phase_voltage_per_switching_state, y_phase_voltage_per_switching_state, id_ref, iq_ref, ix_ref, iy_ref)
     
        % Prediction of the d-, q-, x-, y-currents of the 6-Phase-PMSM with the finite control set 
        id_k_2 = single(SampleTime_div_Ld*(d_phase_voltage_per_switching_state-id_k_1*Rs+omega_el*Lq*iq_k_1)+id_k_1);
        iq_k_2 = single(SampleTime_div_Lq*(q_phase_voltage_per_switching_state-iq_k_1*Rs-omega_el*(psiPM+id_k_1*Ld))+iq_k_1);
        ix_k_2 = single(SampleTime_div_Lx*(x_phase_voltage_per_switching_state-ix_k_1*Rs)+ix_k_1);
        iy_k_2 = single(SampleTime_div_Ly*(y_phase_voltage_per_switching_state-iy_k_1*Rs)+iy_k_1);
        
        % Calculation of the cost function
        J = single((id_ref-id_k_2)^2+(iq_ref-iq_k_2)^2+(ix_ref-ix_k_2)^2+(iy_ref-iy_k_2)^2);
      

end

== matlab function parallel_8_prediction_and_cost_function/Prediction_and_cost_function2/Subsystem/MATLAB Function15 ==
  data: SampleTime_div_Ld input; J output; SampleTime_div_Lq input; SampleTime_div_Lx input; SampleTime_div_Ly input; id_k_1 input; iq_k_1 input; ix_k_1 input; iy_k_1 input; Rs input; omega_el input; Lq input; Ld input; psiPM input; d_phase_voltage_per_switching_state input; q_phase_voltage_per_switching_state input; x_phase_voltage_per_switching_state input; y_phase_voltage_per_switching_state input; id_ref input; iq_ref input; ix_ref input; iy_ref input
function J = fcn(SampleTime_div_Ld, SampleTime_div_Lq, SampleTime_div_Lx, SampleTime_div_Ly, id_k_1, iq_k_1, ix_k_1, iy_k_1, Rs, omega_el, Lq, Ld, psiPM, d_phase_voltage_per_switching_state, q_phase_voltage_per_switching_state, x_phase_voltage_per_switching_state, y_phase_voltage_per_switching_state, id_ref, iq_ref, ix_ref, iy_ref)
     
        % Prediction of the d-, q-, x-, y-currents of the 6-Phase-PMSM with the finite control set 
        id_k_2 = single(SampleTime_div_Ld*(d_phase_voltage_per_switching_state-id_k_1*Rs+omega_el*Lq*iq_k_1)+id_k_1);
        iq_k_2 = single(SampleTime_div_Lq*(q_phase_voltage_per_switching_state-iq_k_1*Rs-omega_el*(psiPM+id_k_1*Ld))+iq_k_1);
        ix_k_2 = single(SampleTime_div_Lx*(x_phase_voltage_per_switching_state-ix_k_1*Rs)+ix_k_1);
        iy_k_2 = single(SampleTime_div_Ly*(y_phase_voltage_per_switching_state-iy_k_1*Rs)+iy_k_1);
        
        % Calculation of the cost function
        J = single((id_ref-id_k_2)^2+(iq_ref-iq_k_2)^2+(ix_ref-ix_k_2)^2+(iy_ref-iy_k_2)^2);

end

== matlab function parallel_8_prediction_and_cost_function/Prediction_and_cost_function2/Subsystem/MATLAB Function8 ==
  data: SampleTime_div_Ld input; J output; SampleTime_div_Lq input; SampleTime_div_Lx input; SampleTime_div_Ly input; id_k_1 input; iq_k_1 input; ix_k_1 input; iy_k_1 input; Rs input; omega_el input; Lq input; Ld input; psiPM input; d_phase_voltage_per_switching_state input; q_phase_voltage_per_switching_state input; x_phase_voltage_per_switching_state input; y_phase_voltage_per_switching_state input; id_ref input; iq_ref input; ix_ref input; iy_ref input
function J = fcn(SampleTime_div_Ld, SampleTime_div_Lq, SampleTime_div_Lx, SampleTime_div_Ly, id_k_1, iq_k_1, ix_k_1, iy_k_1, Rs, omega_el, Lq, Ld, psiPM, d_phase_voltage_per_switching_state, q_phase_voltage_per_switching_state, x_phase_voltage_per_switching_state, y_phase_voltage_per_switching_state, id_ref, iq_ref, ix_ref, iy_ref)
     
        % Prediction of the d-, q-, x-, y-currents of the 6-Phase-PMSM with the finite control set 
        id_k_2 = single(SampleTime_div_Ld*(d_phase_voltage_per_switching_state-id_k_1*Rs+omega_el*Lq*iq_k_1)+id_k_1);
        iq_k_2 = single(SampleTime_div_Lq*(q_phase_voltage_per_switching_state-iq_k_1*Rs-omega_el*(psiPM+id_k_1*Ld))+iq_k_1);
        ix_k_2 = single(SampleTime_div_Lx*(x_phase_voltage_per_switching_state-ix_k_1*Rs)+ix_k_1);
        iy_k_2 = single(SampleTime_div_Ly*(y_phase_voltage_per_switching_state-iy_k_1*Rs)+iy_k_1);
        
        % Calculation of the cost function
        J = single((id_ref-id_k_2)^2+(iq_ref-iq_k_2)^2+(ix_ref-ix_k_2)^2+(iy_ref-iy_k_2)^2);

end

== matlab function parallel_8_prediction_and_cost_function/Prediction_and_cost_function2/Subsystem/MATLAB Function9 ==
  data: SampleTime_div_Ld input; J output; SampleTime_div_Lq input; SampleTime_div_Lx input; SampleTime_div_Ly input; id_k_1 input; iq_k_1 input; ix_k_1 input; iy_k_1 input; Rs input; omega_el input; Lq input; Ld input; psiPM input; d_phase_voltage_per_switching_state input; q_phase_voltage_per_switching_state input; x_phase_voltage_per_switching_state input; y_phase_voltage_per_switching_state input; id_ref input; iq_ref input; ix_ref input; iy_ref input
function J = fcn(SampleTime_div_Ld, SampleTime_div_Lq, SampleTime_div_Lx, SampleTime_div_Ly, id_k_1, iq_k_1, ix_k_1, iy_k_1, Rs, omega_el, Lq, Ld, psiPM, d_phase_voltage_per_switching_state, q_phase_voltage_per_switching_state, x_phase_voltage_per_switching_state, y_phase_voltage_per_switching_state, id_ref, iq_ref, ix_ref, iy_ref)
     
        % Prediction of the d-, q-, x-, y-currents of the 6-Phase-PMSM with the finite control set 
        id_k_2 = single(SampleTime_div_Ld*(d_phase_voltage_per_switching_state-id_k_1*Rs+omega_el*Lq*iq_k_1)+id_k_1);
        iq_k_2 = single(SampleTime_div_Lq*(q_phase_voltage_per_switching_state-iq_k_1*Rs-omega_el*(psiPM+id_k_1*Ld))+iq_k_1);
        ix_k_2 = single(SampleTime_div_Lx*(x_phase_voltage_per_switching_state-ix_k_1*Rs)+ix_k_1);
        iy_k_2 = single(SampleTime_div_Ly*(y_phase_voltage_per_switching_state-iy_k_1*Rs)+iy_k_1);
        
        % Calculation of the cost function
        J = single((id_ref-id_k_2)^2+(iq_ref-iq_k_2)^2+(ix_ref-ix_k_2)^2+(iy_ref-iy_k_2)^2);

end

== matlab function parallel_8_prediction_and_cost_function/Prediction_and_cost_function1/Subsystem/MATLAB Function11 ==
  data: SampleTime_div_Ld input; J output; SampleTime_div_Lq input; SampleTime_div_Lx input; SampleTime_div_Ly input; id_k_1 input; iq_k_1 input; ix_k_1 input; iy_k_1 input; Rs input; omega_el input; Lq input; Ld input; psiPM input; d_phase_voltage_per_switching_state input; q_phase_voltage_per_switching_state input; x_phase_voltage_per_switching_state input; y_phase_voltage_per_switching_state input; id_ref input; iq_ref input; ix_ref input; iy_ref input
function J = fcn(SampleTime_div_Ld, SampleTime_div_Lq, SampleTime_div_Lx, SampleTime_div_Ly, id_k_1, iq_k_1, ix_k_1, iy_k_1, Rs, omega_el, Lq, Ld, psiPM, d_phase_voltage_per_switching_state, q_phase_voltage_per_switching_state, x_phase_voltage_per_switching_state, y_phase_voltage_per_switching_state, id_ref, iq_ref, ix_ref, iy_ref)
     
        % Prediction of the d-, q-, x-, y-currents of the 6-Phase-PMSM with the finite control set 
        id_k_2 = single(SampleTime_div_Ld*(d_phase_voltage_per_switching_state-id_k_1*Rs+omega_el*Lq*iq_k_1)+id_k_1);
        iq_k_2 = single(SampleTime_div_Lq*(q_phase_voltage_per_switching_state-iq_k_1*Rs-omega_el*(psiPM+id_k_1*Ld))+iq_k_1);
        ix_k_2 = single(SampleTime_div_Lx*(x_phase_voltage_per_switching_state-ix_k_1*Rs)+ix_k_1);
        iy_k_2 = single(SampleTime_div_Ly*(y_phase_voltage_per_switching_state-iy_k_1*Rs)+iy_k_1);
        
        % Calculation of the cost function
        J = single((id_ref-id_k_2)^2+(iq_ref-iq_k_2)^2+(ix_ref-ix_k_2)^2+(iy_ref-iy_k_2)^2);

end

== matlab function parallel_8_prediction_and_cost_function/Prediction_and_cost_function1/Subsystem/MATLAB Function12 ==
  data: SampleTime_div_Ld input; J output; SampleTime_div_Lq input; SampleTime_div_Lx input; SampleTime_div_Ly input; id_k_1 input; iq_k_1 input; ix_k_1 input; iy_k_1 input; Rs input; omega_el input; Lq input; Ld input; psiPM input; d_phase_voltage_per_switching_state input; q_phase_voltage_per_switching_state input; x_phase_voltage_per_switching_state input; y_phase_voltage_per_switching_state input; id_ref input; iq_ref input; ix_ref input; iy_ref input
function J = fcn(SampleTime_div_Ld, SampleTime_div_Lq, SampleTime_div_Lx, SampleTime_div_Ly, id_k_1, iq_k_1, ix_k_1, iy_k_1, Rs, omega_el, Lq, Ld, psiPM, d_phase_voltage_per_switching_state, q_phase_voltage_per_switching_state, x_phase_voltage_per_switching_state, y_phase_voltage_per_switching_state, id_ref, iq_ref, ix_ref, iy_ref)
     
        % Prediction of the d-, q-, x-, y-currents of the 6-Phase-PMSM with the finite control set 
        id_k_2 = single(SampleTime_div_Ld*(d_phase_voltage_per_switching_state-id_k_1*Rs+omega_el*Lq*iq_k_1)+id_k_1);
        iq_k_2 = single(SampleTime_div_Lq*(q_phase_voltage_per_switching_state-iq_k_1*Rs-omega_el*(psiPM+id_k_1*Ld))+iq_k_1);
        ix_k_2 = single(SampleTime_div_Lx*(x_phase_voltage_per_switching_state-ix_k_1*Rs)+ix_k_1);
        iy_k_2 = single(SampleTime_div_Ly*(y_phase_voltage_per_switching_state-iy_k_1*Rs)+iy_k_1);
        
        % Calculation of the cost function
        J = single((id_ref-id_k_2)^2+(iq_ref-iq_k_2)^2+(ix_ref-ix_k_2)^2+(iy_ref-iy_k_2)^2);

end
